simulink model "sampleModel2037_3"  (R2023a)
settings: Solver=VariableStepAuto  StartTime=0.0  StopTime=10.0  RelTol=1e-3
libraries: hdlsllib x5
settings Model: Creator=user1  LastModifiedBy=user1

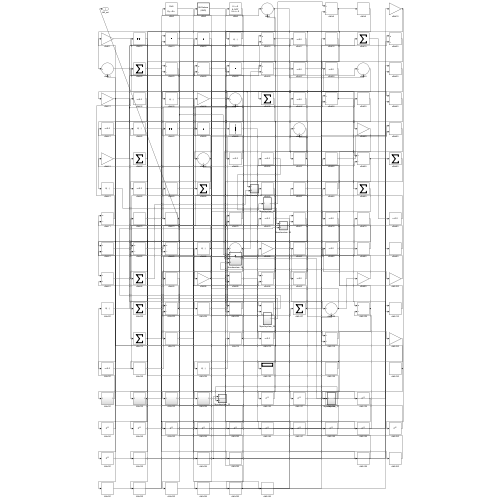
[thumbnail: Simulink's stored preview of the top-level diagram]
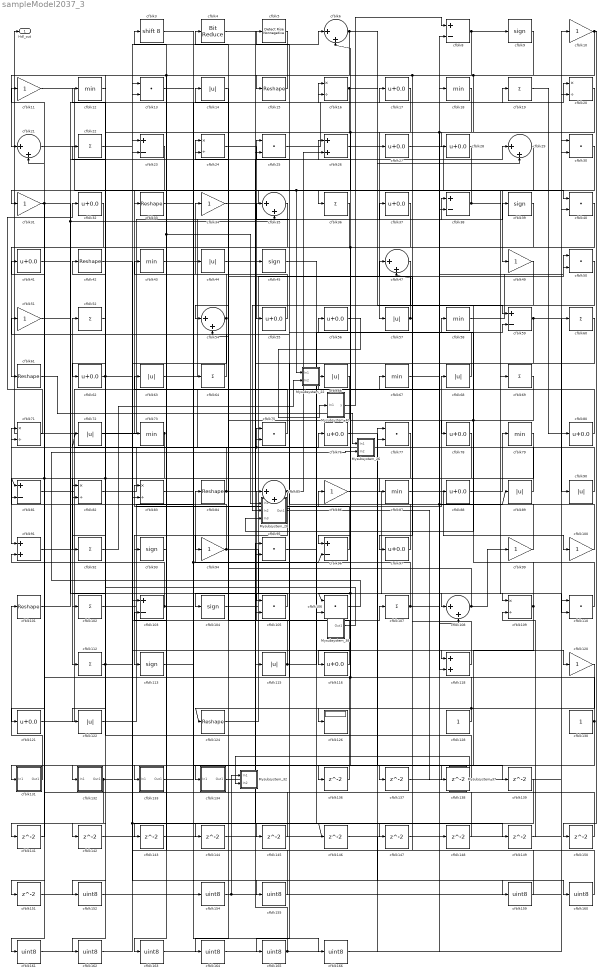
== system sampleModel2037_3 ==
  Mysubsystem_22 : Subsystem  TreatAsAtomicUnit=on  RTWFcnName=Mysubsystem_22
      settings: RTWFcnNameOpts=User specified  RTWFileNameOpts=Use function name
  Mysubsystem_26 : Subsystem  TreatAsAtomicUnit=on  RTWFcnName=Mysubsystem_26
      settings: RTWFcnNameOpts=User specified  RTWFileNameOpts=Use function name
  Mysubsystem_28 : Subsystem  TreatAsAtomicUnit=on  RTWFcnName=Mysubsystem_28
      settings: RTWFcnNameOpts=User specified  RTWFileNameOpts=Use function name
  Mysubsystem_32 : Subsystem  TreatAsAtomicUnit=on  RTWFcnName=Mysubsystem_32
      settings: RTWFcnNameOpts=User specified  RTWFileNameOpts=Use function name
  Mysubsystem_37 : Subsystem  TreatAsAtomicUnit=on  RTWFcnName=Mysubsystem_37
      settings: RTWFcnNameOpts=User specified  RTWFileNameOpts=Use function name
  Mysubsystem_38 : Subsystem  TreatAsAtomicUnit=on  RTWFcnName=Mysubsystem_38
      settings: RTWFcnNameOpts=User specified  RTWFileNameOpts=Use function name
  Mysubsystem_40 : Subsystem  TreatAsAtomicUnit=on  RTWFcnName=Mysubsystem_40
      settings: RTWFcnNameOpts=User specified  RTWFileNameOpts=Use function name
  cfblk{10..11,31,34,49,51,86,94,99..100,120} (11 alike) : Gain  OutDataTypeStr=uint8
  cfblk{15,33,42,61,84,101,124} (7 alike) : Reshape
  cfblk{19,22,36,52,60,64,69,92,102,107,112} (11 alike) : Sum  Inputs=+  OutDataTypeStr=uint8
  cfblk{8,23,38,59,81,96,103} (7 alike) : Sum  Inputs=+-  OutDataTypeStr=uint8
  cfblk{9,39,45,93,104,113} (6 alike) : Signum
  cfblk{13,25,30,40,50,75,77,95,105..106,110} (11 alike) : DotProduct  OutDataTypeStr=uint8
  cfblk{6,21,29,35,47,54,85,108} (8 alike) : Sum  Inputs=|++  OutDataTypeStr=uint8
  cfblk{16,20,24,71,82..83,109} (7 alike) : Product  Inputs=*/  OutDataTypeStr=uint8  RndMeth=Zero  SaturateOnIntegerOverflow=on
  cfblk{14,44,57,63,66,68,72,89..90,115,122} (11 alike) : Abs  OutDataTypeStr=uint8  SaturateOnIntegerOverflow=off
  cfblk{17,27..28,32,37,41,55..56,62,76,78,80,88,97,116,121} (16 alike) : Bias  Bias=0.0  SaturateOnIntegerOverflow=off
  cfblk118 : Sum  OutDataTypeStr=uint8
  cfblk{12,18,43,58,67,73,79,87} (8 alike) : MinMax  OutDataTypeStr=uint8
  cfblk126 : Display
  cfblk128 : Constant  OutDataTypeStr=uint8  SampleTime=-1
  cfblk130 : Constant  OutDataTypeStr=uint8  SampleTime=-1
  cfblk131 : Subsystem
      settings: LibrarySourceBlock=|
      | hdlsllib/Ports &
      | Subsystems/Subsystem
  cfblk132 : Subsystem
      settings: LibrarySourceBlock=|
      | hdlsllib/Ports &
      | Subsystems/Subsystem
  cfblk133 : Subsystem
      settings: LibrarySourceBlock=|
      | hdlsllib/Ports &
      | Subsystems/Subsystem
  cfblk134 : Subsystem
      settings: LibrarySourceBlock=|
      | hdlsllib/Ports &
      | Subsystems/Subsystem
  cfblk{136..139,141..151} (15 alike) : Delay  SampleTime=1
  cfblk{152,154..155,159..166} (11 alike) : DataTypeConversion  OutDataTypeStr=uint8  SaturateOnIntegerOverflow=off  RndMeth=Floor
  cfblk26 : Sum  OutDataTypeStr=uint8
  cfblk3 : ArithShift  BitShiftNumber=8
  cfblk4 : hdlsllib/Logic and Bit Operations/Bit Reduce  mode=AND
  cfblk5 : hdlsllib/Logic and Bit Operations/Detect Rise Nonnegative  vinit=0  OutDataTypeStr=uint8
  cfblk91 : Sum  OutDataTypeStr=uint8
  Hdl_out : Outport  OutDataTypeStr=uint8
  wires:
  cfblk105/1 -> cfblk104/1
  cfblk72/1 -> cfblk38/1
  cfblk122/1 -> cfblk86/1
  cfblk11/1 -> cfblk49/1
  cfblk36/1 -> cfblk61/1
  cfblk17/1 -> cfblk57/1
  cfblk19/1 -> cfblk80/1
  cfblk63/1 -> cfblk37/1
  cfblk66/1 -> cfblk134/1(In1)
  cfblk71/1 -> cfblk32/1
  cfblk23/1 -> cfblk73/1
  cfblk131/1(Out1) -> cfblk101/1
  cfblk108/1 -> cfblk99/1, cfblk54/2
  cfblk121/1 -> cfblk66/1
  cfblk112/1 -> cfblk12/1, cfblk118/1
  cfblk43/1 -> cfblk39/1
  cfblk15/1 -> cfblk21/1
  cfblk104/1 -> cfblk76/1
  cfblk99/1 -> cfblk51/1
  cfblk97/1 -> cfblk5/1
  cfblk79/1 -> cfblk112/1
  cfblk124/1 -> cfblk50/1
  cfblk90/1 -> cfblk56/1
  cfblk100/1 -> cfblk68/1
  cfblk26/1 -> cfblk27/1
  cfblk69/1 -> Mysubsystem_28/3(In3), cfblk126/1, cfblk106/1
  cfblk93/1 -> cfblk133/1(In1)
  cfblk27/1 -> cfblk69/1
  cfblk116/1 -> cfblk24/1
  cfblk49/1 -> cfblk78/1
  cfblk91/1 -> cfblk52/1
  cfblk42/1 -> cfblk146/1, cfblk155/1
  cfblk118/1 -> cfblk47/1
  cfblk86/1 -> cfblk109/1
  cfblk18/1 -> cfblk62/1, cfblk118/2
  cfblk60/1 -> cfblk165/1
  cfblk134/1(Out1) -> cfblk115/1
  cfblk55/1 -> cfblk34/1
  cfblk81/1 -> cfblk18/1
  cfblk89/1 -> cfblk14/1
  cfblk38/1 -> cfblk31/1, cfblk110/2
  cfblk24/1 -> cfblk55/1
  cfblk6/1 -> cfblk15/1, cfblk59/1
  cfblk34/1 -> cfblk40/1
  cfblk80/1 -> cfblk25/1
  cfblk94/1 -> cfblk71/1, cfblk106/2
  cfblk85/1 -> cfblk113/1, cfblk26/2
  cfblk110/1 -> cfblk58/1
  cfblk133/1(Out1) -> cfblk20/1, cfblk96/2
  cfblk5/1 -> cfblk102/1
  cfblk109/1 -> cfblk75/1, cfblk72/1, cfblk138/1
  cfblk54/1 -> cfblk43/1, cfblk83/2
  cfblk64/1 -> cfblk42/1
  cfblk87/1 -> cfblk100/1
  cfblk57/1 -> cfblk97/1, cfblk4/1
  cfblk30/1 -> cfblk45/1
  cfblk47/1 -> cfblk116/1
  cfblk107/1 -> cfblk89/1, cfblk50/2, cfblk84/1
  cfblk35/1 -> cfblk122/1
  cfblk20/1 -> cfblk94/1, cfblk36/1
  cfblk21/1 -> cfblk24/2
  cfblk9/1 -> cfblk47/2, cfblk25/2, cfblk28/1
  cfblk25/1 -> cfblk17/1
  cfblk128/1 -> cfblk85/2, cfblk6/2, cfblk124/1
  cfblk82/1 -> cfblk44/1
  cfblk62/1 -> cfblk23/2, cfblk92/1
  cfblk88/1 -> cfblk79/1
  cfblk130/1 -> cfblk41/1, cfblk131/1(In1)
  cfblk40/1 -> cfblk54/1, cfblk136/1
  cfblk113/1 -> cfblk75/2
  cfblk115/1 -> cfblk85/1, cfblk59/2
  cfblk96/1 -> cfblk83/1
  cfblk132/1(Out1) -> cfblk107/1, cfblk161/1
  cfblk73/1 -> cfblk91/1, Hdl_out/1
  cfblk12/1 -> cfblk82/1
  cfblk78/1 -> cfblk141/1, cfblk142/1
  cfblk103/1 -> cfblk88/1, cfblk81/2
  cfblk59/1 -> cfblk90/1, cfblk105/2
  cfblk102/1 -> cfblk64/1
  cfblk22/1 -> cfblk6/1
  cfblk45/1 -> cfblk120/1
  cfblk68/1 -> cfblk35/1
  cfblk44/1 -> cfblk108/1
  cfblk32/1 -> cfblk81/1, cfblk151/1
  cfblk84/1 -> cfblk11/1, cfblk29/1
  cfblk101/1 -> cfblk26/1
  cfblk10/1 -> cfblk132/1(In1), cfblk33/1, cfblk150/1
  cfblk39/1 -> cfblk87/1
  cfblk31/1 -> cfblk105/1, cfblk121/1
  cfblk67/1 -> cfblk19/1
  cfblk52/1 -> cfblk22/1
  cfblk58/1 -> cfblk10/1
  cfblk75/1 -> cfblk63/1
  cfblk41/1 -> cfblk35/2, cfblk16/2
  cfblk8/1 -> cfblk9/1, cfblk95/2
  cfblk51/1 -> cfblk16/1
  cfblk16/1 -> cfblk93/1, cfblk29/2
  cfblk37/1 -> cfblk96/1
  cfblk29/1 -> Mysubsystem_22/1(In1), Mysubsystem_28/1(In1), cfblk143/1
  cfblk136/1 -> cfblk71/2
  cfblk83/1 -> cfblk137/1
  cfblk137/1 -> cfblk40/2
  cfblk138/1 -> cfblk82/2
  cfblk76/1 -> cfblk139/1
  cfblk141/1 -> cfblk21/2
  cfblk142/1 -> cfblk20/2
  cfblk143/1 -> cfblk110/1
  cfblk14/1 -> cfblk144/1
  cfblk144/1 -> cfblk38/2
  cfblk120/1 -> cfblk145/1
  cfblk145/1 -> cfblk91/2
  cfblk4/1 -> cfblk147/1
  cfblk147/1 -> cfblk8/2
  cfblk148/1 -> cfblk23/1
  cfblk95/1 -> cfblk149/1
  cfblk149/1 -> cfblk109/2
  cfblk150/1 -> cfblk103/2
  cfblk151/1 -> cfblk108/2
  cfblk152/1 -> Mysubsystem_32/1(In1), cfblk30/2
  cfblk3/1 -> cfblk154/1
  cfblk154/1 -> cfblk30/1
  cfblk155/1 -> cfblk3/1
  cfblk13/1 -> cfblk159/1
  cfblk159/1 -> cfblk67/1
  cfblk146/1 -> cfblk160/1
  cfblk160/1 -> cfblk13/1
  cfblk161/1 -> cfblk13/2
  cfblk77/1 -> cfblk162/1
  cfblk162/1 -> cfblk103/1
  cfblk139/1 -> cfblk163/1
  cfblk163/1 -> cfblk77/1
  cfblk28/1 -> cfblk164/1
  cfblk164/1 -> cfblk77/2
  cfblk165/1 -> cfblk148/1, cfblk95/1
  cfblk33/1 -> cfblk166/1
  cfblk166/1 -> cfblk60/1
  cfblk92/1 -> Mysubsystem_22/2(In2)
  cfblk61/1 -> Mysubsystem_26/1(In1)
  cfblk106/1 -> Mysubsystem_26/2(In2)
  cfblk50/1 -> Mysubsystem_28/2(In2)
  Mysubsystem_28/1(Out1) -> Mysubsystem_37/1(In1)
  Mysubsystem_37/1(Out1) -> Mysubsystem_32/2(In2)
  Mysubsystem_38/1(Out1) -> cfblk152/1
  cfblk56/1 -> Mysubsystem_40/1(In1)
  Mysubsystem_40/1(y) -> cfblk8/1

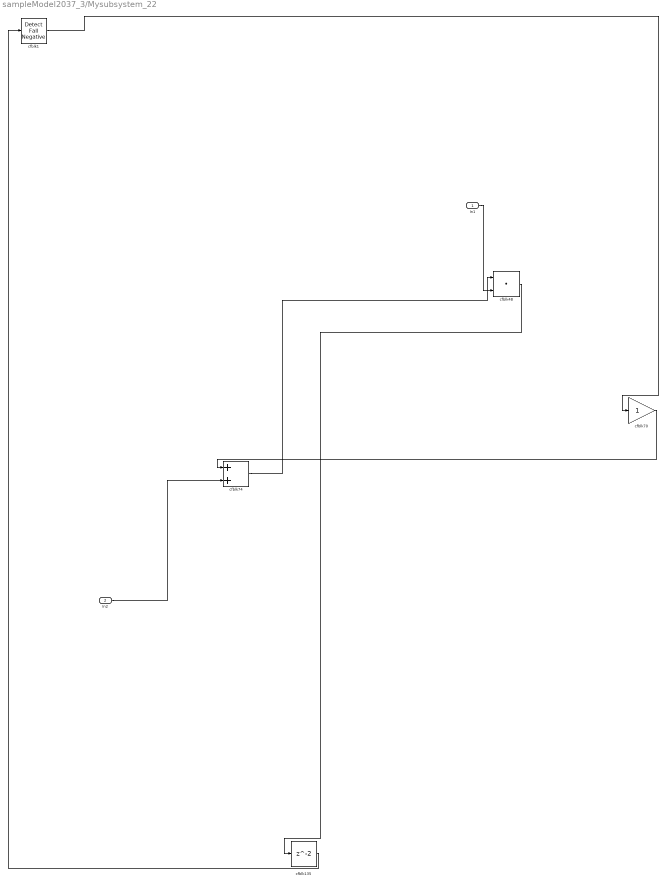
== system sampleModel2037_3/Mysubsystem_22 ==
  In1 : Inport
  In2 : Inport  Port=2
  cfblk1 : hdlsllib/Logic and Bit Operations/Detect Fall Negative  vinit=0  OutDataTypeStr=boolean
  cfblk135 : Delay  SampleTime=1
  cfblk48 : DotProduct  OutDataTypeStr=Inherit: Inherit via internal rule
  cfblk70 : Gain
  cfblk74 : Sum
  wires:
  cfblk74/1 -> cfblk48/1
  cfblk1/1 -> cfblk70/1
  In2/1 -> cfblk74/2
  cfblk70/1 -> cfblk74/1
  cfblk135/1 -> cfblk1/1
  In1/1 -> cfblk48/2
  cfblk48/1 -> cfblk135/1

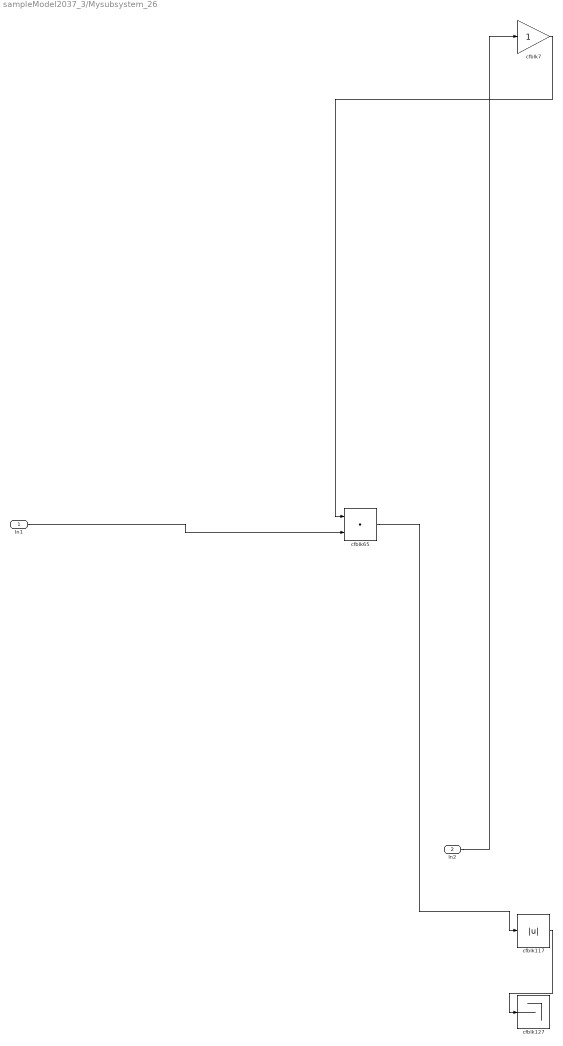
== system sampleModel2037_3/Mysubsystem_26 ==
  In1 : Inport
  In2 : Inport  Port=2
  cfblk117 : Abs  SaturateOnIntegerOverflow=off
  cfblk127 : Terminator
  cfblk65 : DotProduct  OutDataTypeStr=Inherit: Inherit via internal rule
  cfblk7 : Gain
  wires:
  In1/1 -> cfblk65/2
  cfblk65/1 -> cfblk117/1
  cfblk7/1 -> cfblk65/1
  cfblk117/1 -> cfblk127/1
  In2/1 -> cfblk7/1

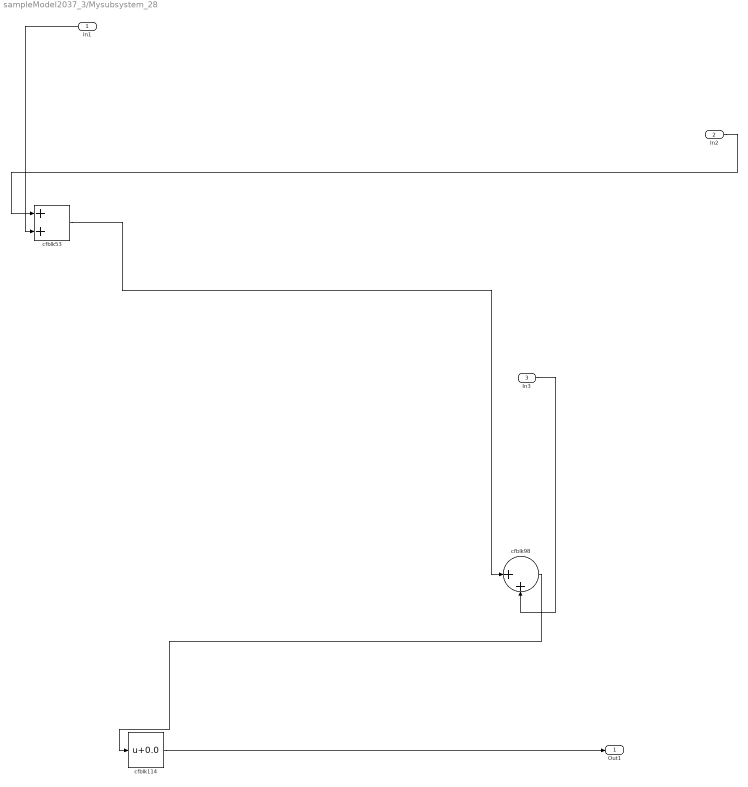
== system sampleModel2037_3/Mysubsystem_28 ==
  In1 : Inport
  In2 : Inport  Port=2
  In3 : Inport  Port=3
  cfblk114 : Bias  Bias=0.0  SaturateOnIntegerOverflow=off
  cfblk53 : Sum
  cfblk98 : Sum  Inputs=|++
  Out1 : Outport
  wires:
  cfblk53/1 -> cfblk98/1
  cfblk98/1 -> cfblk114/1
  In2/1 -> cfblk53/1
  cfblk114/1 -> Out1/1
  In3/1 -> cfblk98/2
  In1/1 -> cfblk53/2

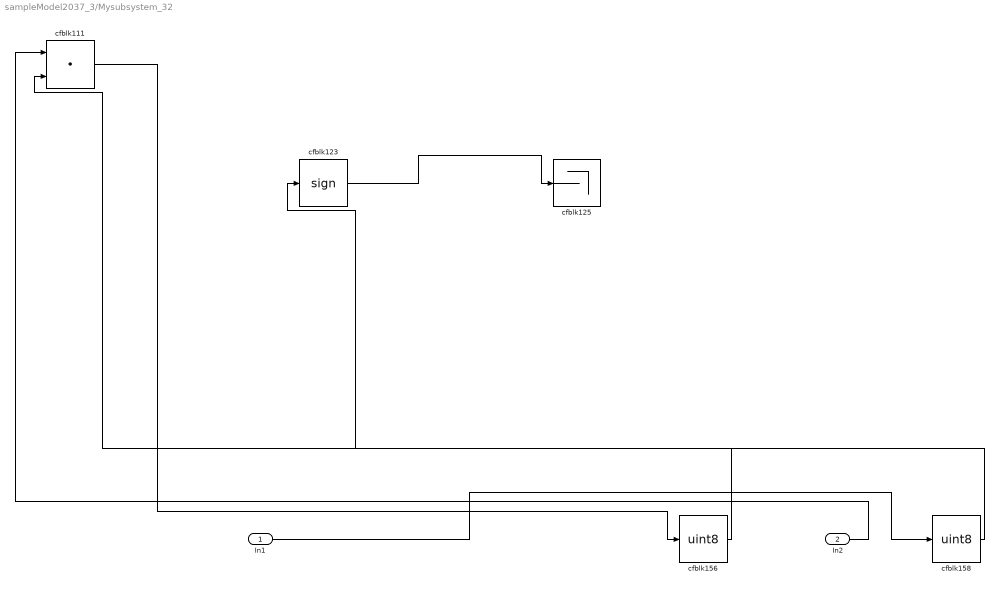
== system sampleModel2037_3/Mysubsystem_32 ==
  In1 : Inport
  In2 : Inport  Port=2
  cfblk111 : DotProduct  OutDataTypeStr=Inherit: Inherit via internal rule
  cfblk123 : Signum
  cfblk125 : Terminator
  cfblk156 : DataTypeConversion  OutDataTypeStr=uint8  SaturateOnIntegerOverflow=off  RndMeth=Floor
  cfblk158 : DataTypeConversion  OutDataTypeStr=uint8  SaturateOnIntegerOverflow=off  RndMeth=Floor
  wires:
  cfblk123/1 -> cfblk125/1
  cfblk158/1 -> cfblk111/2
  cfblk111/1 -> cfblk156/1
  In1/1 -> cfblk158/1
  cfblk156/1 -> cfblk123/1
  In2/1 -> cfblk111/1

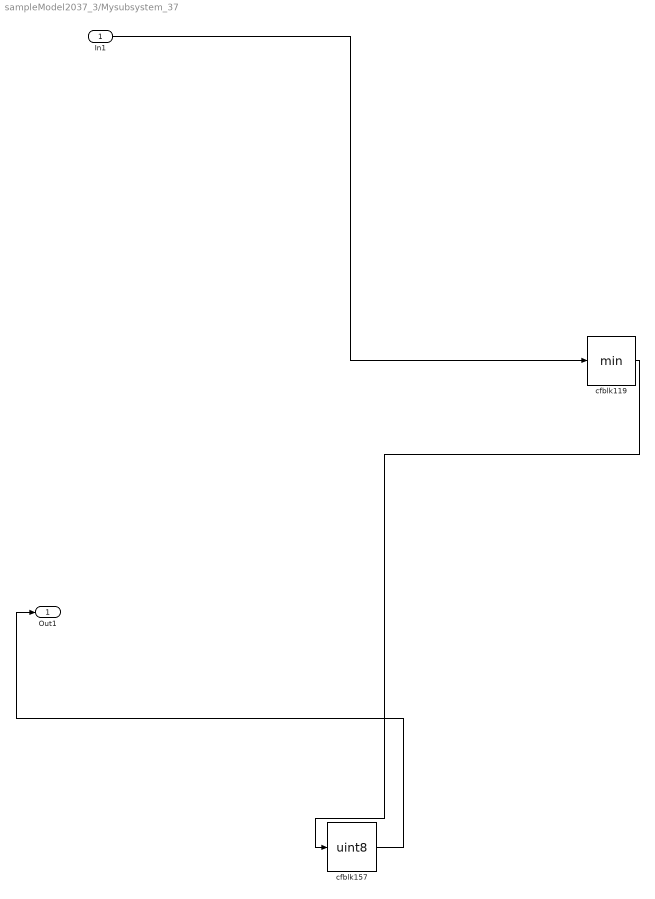
== system sampleModel2037_3/Mysubsystem_37 ==
  In1 : Inport
  cfblk119 : MinMax
  cfblk157 : DataTypeConversion  OutDataTypeStr=uint8  SaturateOnIntegerOverflow=off  RndMeth=Floor
  Out1 : Outport
  wires:
  cfblk119/1 -> cfblk157/1
  In1/1 -> cfblk119/1
  cfblk157/1 -> Out1/1

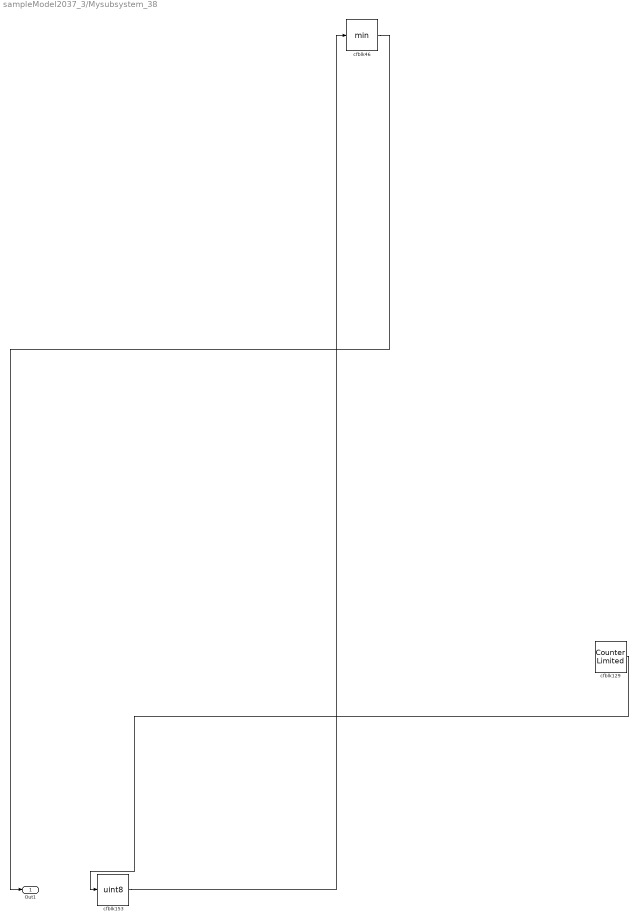
== system sampleModel2037_3/Mysubsystem_38 ==
  cfblk129 : hdlsllib/Sources/Counter Limited  uplimit=7  tsamp=-1
  cfblk153 : DataTypeConversion  OutDataTypeStr=uint8  SaturateOnIntegerOverflow=off  RndMeth=Floor
  cfblk46 : MinMax
  Out1 : Outport
  wires:
  cfblk129/1 -> cfblk153/1
  cfblk46/1 -> Out1/1
  cfblk153/1 -> cfblk46/1

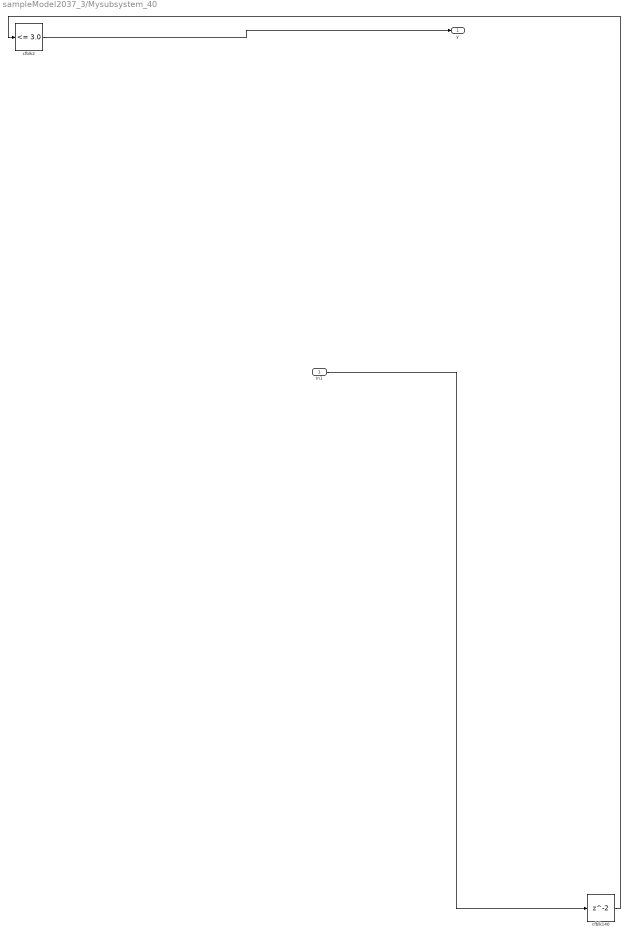
== system sampleModel2037_3/Mysubsystem_40 ==
  In1 : Inport
  cfblk140 : Delay  SampleTime=1
  cfblk2 : hdlsllib/Logic and Bit Operations/Compare To Constant  relop=<=  const=3.0  OutDataTypeStr=boolean
  y : Outport
  wires:
  cfblk140/1 -> cfblk2/1
  cfblk2/1 -> y/1
  In1/1 -> cfblk140/1

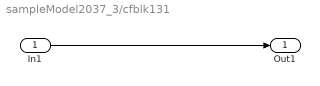
== system sampleModel2037_3/cfblk131 ==
  In1 : Inport
  Out1 : Outport
  wires:
  In1/1 -> Out1/1

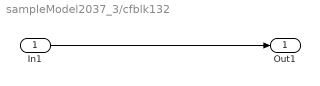
== system sampleModel2037_3/cfblk132 ==
  In1 : Inport
  Out1 : Outport
  wires:
  In1/1 -> Out1/1

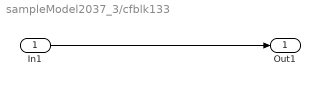
== system sampleModel2037_3/cfblk133 ==
  In1 : Inport
  Out1 : Outport
  wires:
  In1/1 -> Out1/1

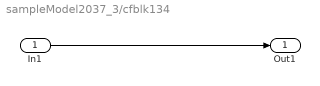
== system sampleModel2037_3/cfblk134 ==
  In1 : Inport
  Out1 : Outport
  wires:
  In1/1 -> Out1/1
